simulink library "VMM_lib"  (Simulink 7.5)
settings: Solver=ode45  StartTime=0.0  StopTime=10.0  RelTol=1e-3
values from neighbouring files (symbols this model uses):
  pVMM_kmph_VehLgtSpdThd_C = Simulink.Parameter    [VMM_par.m]
  pVMM_s_EparkCheckTiOut_C = Simulink.Parameter    [VMM_par.m]
  pVMM_s_EparkShutdownTiOut_C = Simulink.Parameter    [VMM_par.m]
  pVMM_s_ShtdwnAckDly_C = Simulink.Parameter    [VMM_par.m]
  pVMM_s_ThermoShutdownTiOut_C = Simulink.Parameter    [VMM_par.m]
libraries: BaseOperationLib_Browser x15, PES_CZ_FAW x15, simulink x1
settings Model: Creator=wuaibin  LastModifiedBy=wuaibin

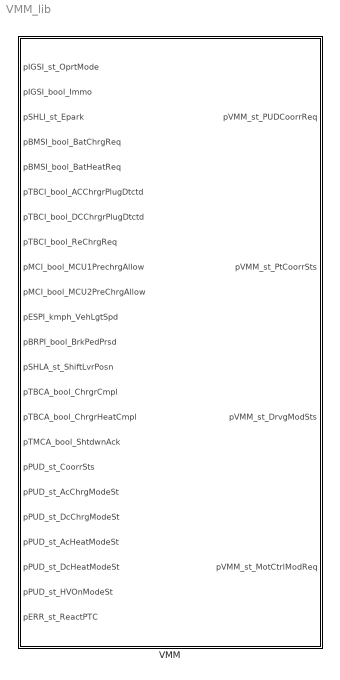
== system VMM_lib ==
  VMM : Subsystem  TreatAsAtomicUnit=on

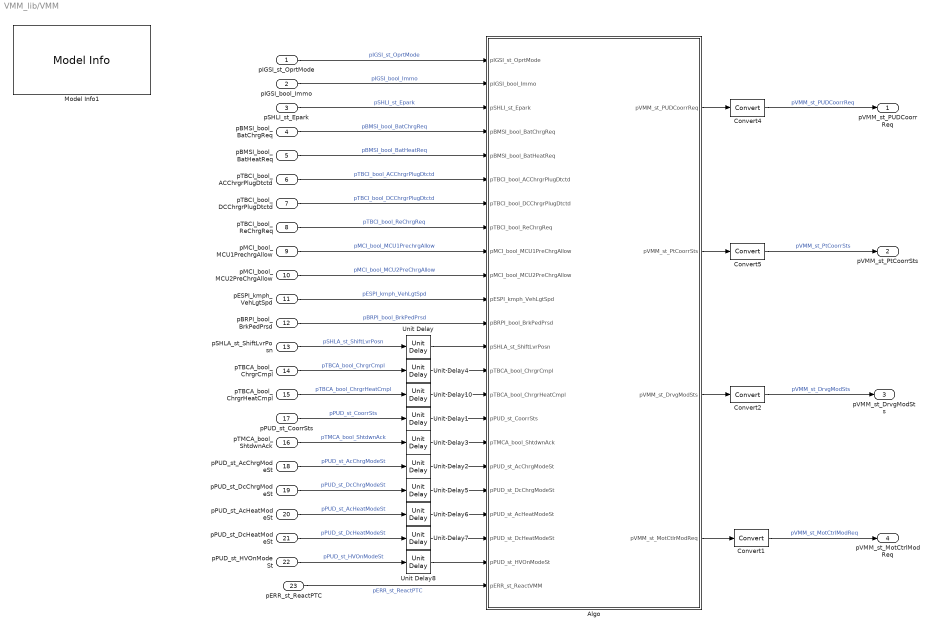
== system VMM_lib/VMM ==
  pIGSI_st_OprtMode : Inport
  pIGSI_bool_Immo : Inport  Port=2
  pSHLI_st_Epark : Inport  Port=3
  pBMSI_bool_BatChrgReq : Inport  Port=4
  pBMSI_bool_BatHeatReq : Inport  Port=5
  pTBCI_bool_ACChrgrPlugDtctd : Inport  Port=6
  pTBCI_bool_DCChrgrPlugDtctd : Inport  Port=7
  pTBCI_bool_ReChrgReq : Inport  Port=8
  pMCI_bool_MCU1PrechrgAllow : Inport  Port=9
  pMCI_bool_MCU2PreChrgAllow : Inport  Port=10
  pESPI_kmph_VehLgtSpd : Inport  Port=11
  pBRPI_bool_BrkPedPrsd : Inport  Port=12
  pSHLA_st_ShiftLvrPosn : Inport  Port=13
  pTBCA_bool_ChrgrCmpl : Inport  Port=14
  pTBCA_bool_ChrgrHeatCmpl : Inport  Port=15
  pTMCA_bool_ShtdwnAck : Inport  Port=16
  pPUD_st_CoorrSts : Inport  Port=17
  pPUD_st_AcChrgModeSt : Inport  Port=18
  pPUD_st_DcChrgModeSt : Inport  Port=19
  pPUD_st_AcHeatModeSt : Inport  Port=20
  pPUD_st_DcHeatModeSt : Inport  Port=21
  pPUD_st_HVOnModeSt : Inport  Port=22
  pERR_st_ReactPTC : Inport  Port=23
  Algo : Subsystem
  Convert{1..2,4..5} (4 alike) : DataTypeConversion  OutDataType=fixdt(1, 16)  OutScaling=2^0
  Model Info1 : simulink/Model-Wide Utilities/Model Info  SystemSampleTime=-1  InitialBlockCM=None  BlockCM=None  Frame=on  DisplayStringWithTags=Model Info\nCreated: %<Created>\nCreator: wuaibin  HorizontalTextAlignment=Center  LeftAlignmentValue=0.5  SourceBlockDiagram=untitled  TagMaxNumber=20
  Unit Delay{,1..8,10} (10 alike) : BaseOperationLib_Browser/Discrete Unchanged /Unit Delay  X0=0  SampleTime=-1
  pVMM_st_PUDCoorrReq : Outport
  pVMM_st_PtCoorrSts : Outport  Port=2
  pVMM_st_DrvgModSts : Outport  Port=3
  pVMM_st_MotCtrlModReq : Outport  Port=4
  wires:
  pTBCI_bool_ReChrgReq/1 -> Algo/8(pTBCI_bool_ReChrgReq)  "pTBCI_bool_ReChrgReq"
  Unit Delay10/1 -> Algo/15(pTBCA_bool_ChrgrHeatCmpl)
  pTBCA_bool_ChrgrHeatCmpl/1 -> Unit Delay10/1  "pTBCA_bool_ChrgrHeatCmpl"
  pMCI_bool_MCU2PreChrgAllow/1 -> Algo/10(pMCI_bool_MCU2PreChrgAllow)  "pMCI_bool_MCU2PreChrgAllow"
  Algo/4(pVMM_st_MotCtlrModReq) -> Convert1/1
  Convert1/1 -> pVMM_st_MotCtrlModReq/1  "pVMM_st_MotCtrlModReq"
  pMCI_bool_MCU1PrechrgAllow/1 -> Algo/9(pMCI_bool_MCU1PreChrgAllow)  "pMCI_bool_MCU1PrechrgAllow"
  Algo/1(pVMM_st_PUDCoorrReq) -> Convert4/1
  Algo/2(pVMM_st_PtCoorrSts) -> Convert5/1
  Algo/3(pVMM_st_DrvgModSts) -> Convert2/1
  pERR_st_ReactPTC/1 -> Algo/23(pERR_st_ReactVMM)  "pERR_st_ReactPTC"
  Unit Delay8/1 -> Algo/22(pPUD_st_HVOnModeSt)
  Unit Delay7/1 -> Algo/21(pPUD_st_DcHeatModeSt)
  Unit Delay6/1 -> Algo/20(pPUD_st_AcHeatModeSt)
  Unit Delay5/1 -> Algo/19(pPUD_st_DcChrgModeSt)
  Unit Delay2/1 -> Algo/18(pPUD_st_AcChrgModeSt)
  Unit Delay3/1 -> Algo/17(pTMCA_bool_ShtdwnAck)
  Unit Delay1/1 -> Algo/16(pPUD_st_CoorrSts)
  Unit Delay4/1 -> Algo/14(pTBCA_bool_ChrgrCmpl)
  Unit Delay/1 -> Algo/13(pSHLA_st_ShiftLvrPosn)
  pBRPI_bool_BrkPedPrsd/1 -> Algo/12(pBRPI_bool_BrkPedPrsd)  "pBRPI_bool_BrkPedPrsd"
  pESPI_kmph_VehLgtSpd/1 -> Algo/11(pESPI_kmph_VehLgtSpd)  "pESPI_kmph_VehLgtSpd"
  pTBCI_bool_DCChrgrPlugDtctd/1 -> Algo/7(pTBCI_bool_DCChrgrPlugDtctd)  "pTBCI_bool_DCChrgrPlugDtctd"
  pTBCI_bool_ACChrgrPlugDtctd/1 -> Algo/6(pTBCI_bool_ACChrgrPlugDtctd)  "pTBCI_bool_ACChrgrPlugDtctd"
  pBMSI_bool_BatHeatReq/1 -> Algo/5(pBMSI_bool_BatHeatReq)  "pBMSI_bool_BatHeatReq"
  pBMSI_bool_BatChrgReq/1 -> Algo/4(pBMSI_bool_BatChrgReq)  "pBMSI_bool_BatChrgReq"
  pSHLI_st_Epark/1 -> Algo/3(pSHLI_st_Epark)  "pSHLI_st_Epark"
  pIGSI_bool_Immo/1 -> Algo/2(pIGSI_bool_Immo)  "pIGSI_bool_Immo"
  pIGSI_st_OprtMode/1 -> Algo/1(pIGSI_st_OprtMode)  "pIGSI_st_OprtMode"
  Convert2/1 -> pVMM_st_DrvgModSts/1  "pVMM_st_DrvgModSts"
  pPUD_st_HVOnModeSt/1 -> Unit Delay8/1  "pPUD_st_HVOnModeSt"
  pPUD_st_DcHeatModeSt/1 -> Unit Delay7/1  "pPUD_st_DcHeatModeSt"
  pPUD_st_AcHeatModeSt/1 -> Unit Delay6/1  "pPUD_st_AcHeatModeSt"
  pPUD_st_DcChrgModeSt/1 -> Unit Delay5/1  "pPUD_st_DcChrgModeSt"
  pPUD_st_AcChrgModeSt/1 -> Unit Delay2/1  "pPUD_st_AcChrgModeSt"
  pTBCA_bool_ChrgrCmpl/1 -> Unit Delay4/1  "pTBCA_bool_ChrgrCmpl"
  pTMCA_bool_ShtdwnAck/1 -> Unit Delay3/1  "pTMCA_bool_ShtdwnAck"
  Convert5/1 -> pVMM_st_PtCoorrSts/1  "pVMM_st_PtCoorrSts"
  Convert4/1 -> pVMM_st_PUDCoorrReq/1  "pVMM_st_PUDCoorrReq"
  pPUD_st_CoorrSts/1 -> Unit Delay1/1  "pPUD_st_CoorrSts"
  pSHLA_st_ShiftLvrPosn/1 -> Unit Delay/1  "pSHLA_st_ShiftLvrPosn"

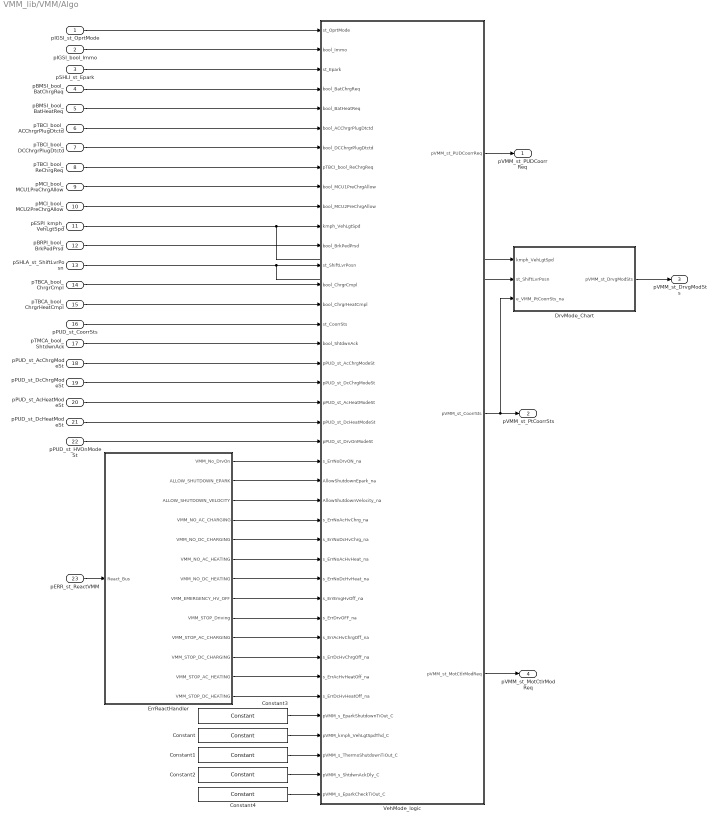
== system VMM_lib/VMM/Algo ==
  pIGSI_st_OprtMode : Inport
  pIGSI_bool_Immo : Inport  Port=2
  pSHLI_st_Epark : Inport  Port=3
  pBMSI_bool_BatChrgReq : Inport  Port=4
  pBMSI_bool_BatHeatReq : Inport  Port=5
  pTBCI_bool_ACChrgrPlugDtctd : Inport  Port=6
  pTBCI_bool_DCChrgrPlugDtctd : Inport  Port=7
  pTBCI_bool_ReChrgReq : Inport  Port=8
  pMCI_bool_MCU1PreChrgAllow : Inport  Port=9
  pMCI_bool_MCU2PreChrgAllow : Inport  Port=10
  pESPI_kmph_VehLgtSpd : Inport  Port=11
  pBRPI_bool_BrkPedPrsd : Inport  Port=12
  pSHLA_st_ShiftLvrPosn : Inport  Port=13
  pTBCA_bool_ChrgrCmpl : Inport  Port=14
  pTBCA_bool_ChrgrHeatCmpl : Inport  Port=15
  pPUD_st_CoorrSts : Inport  Port=16
  pTMCA_bool_ShtdwnAck : Inport  Port=17
  pPUD_st_AcChrgModeSt : Inport  Port=18
  pPUD_st_DcChrgModeSt : Inport  Port=19
  pPUD_st_AcHeatModeSt : Inport  Port=20
  pPUD_st_DcHeatModeSt : Inport  Port=21
  pPUD_st_HVOnModeSt : Inport  Port=22
  pERR_st_ReactVMM : Inport  Port=23
  Constant : BaseOperationLib_Browser/Sources&Sinks/Constant  Value=pVMM_kmph_VehLgtSpdThd_C  OutMin=[]  OutMax=[]  OutDataType=fixdt(1, 16)  ConRadixGroup=Use specified scaling  OutScaling=2^0  OutDataTypeStr=Inherit: Inherit from 'Constant value'
  Constant1 : BaseOperationLib_Browser/Sources&Sinks/Constant  Value=pVMM_s_ThermoShutdownTiOut_C  OutMin=[]  OutMax=[]  OutDataType=fixdt(1, 16)  ConRadixGroup=Use specified scaling  OutScaling=2^0  OutDataTypeStr=Inherit: Inherit from 'Constant value'
  Constant2 : BaseOperationLib_Browser/Sources&Sinks/Constant  Value=pVMM_s_ShtdwnAckDly_C  OutMin=[]  OutMax=[]  OutDataType=fixdt(1, 16)  ConRadixGroup=Use specified scaling  OutScaling=2^0  OutDataTypeStr=Inherit: Inherit from 'Constant value'
  Constant3 : BaseOperationLib_Browser/Sources&Sinks/Constant  Value=pVMM_s_EparkShutdownTiOut_C  OutMin=[]  OutMax=[]  OutDataType=fixdt(1, 16)  ConRadixGroup=Use specified scaling  OutScaling=2^0  OutDataTypeStr=Inherit: Inherit from 'Constant value'
  Constant4 : BaseOperationLib_Browser/Sources&Sinks/Constant  Value=pVMM_s_EparkCheckTiOut_C  OutMin=[]  OutMax=[]  OutDataType=fixdt(1, 16)  ConRadixGroup=Use specified scaling  OutScaling=2^0  OutDataTypeStr=Inherit: Inherit from 'Constant value'
  DrvMode_Chart : Stateflow chart  TreatAsAtomicUnit=on
  ErrReactHandler : Subsystem
  VehMode_logic : Stateflow chart  TreatAsAtomicUnit=on
  pVMM_st_PUDCoorrReq : Outport
  pVMM_st_PtCoorrSts : Outport  Port=2
  pVMM_st_DrvgModSts : Outport  Port=3
  pVMM_st_MotCtlrModReq : Outport  Port=4
  wires:
  Constant2/1 -> VehMode_logic/39(pVMM_s_ShtdwnAckDly_C)
  Constant1/1 -> VehMode_logic/38(pVMM_s_ThermoShutdownTiOut_C)
  Constant3/1 -> VehMode_logic/36(pVMM_s_EparkShutdownTiOut_C)
  Constant/1 -> VehMode_logic/37(pVMM_kmph_VehLgtSpdThd_C)
  pTBCI_bool_ReChrgReq/1 -> VehMode_logic/8(pTBCI_bool_ReChrgReq)
  pMCI_bool_MCU2PreChrgAllow/1 -> VehMode_logic/10(bool_MCU2PreChrgAllow)
  ErrReactHandler/13(VMM_STOP_DC_HEATING) -> VehMode_logic/35(s_ErrDcHvHeatOff_na)
  ErrReactHandler/12(VMM_STOP_AC_HEATING) -> VehMode_logic/34(s_ErrAcHvHeatOff_na)
  ErrReactHandler/11(VMM_STOP_DC_CHARGING) -> VehMode_logic/33(s_ErrDcHvChrgOff_na)
  ErrReactHandler/10(VMM_STOP_AC_CHARGING) -> VehMode_logic/32(s_ErrAcHvChrgOff_na)
  ErrReactHandler/9(VMM_STOP_Driving) -> VehMode_logic/31(s_ErrDrvOFF_na)
  VehMode_logic/2(pVMM_st_CoorrSts) -> DrvMode_Chart/3(e_VMM_PtCoorrSts_na), pVMM_st_PtCoorrSts/1
  pTBCA_bool_ChrgrHeatCmpl/1 -> VehMode_logic/15(bool_ChrgrHeatCmpl)
  pMCI_bool_MCU1PreChrgAllow/1 -> VehMode_logic/9(bool_MCU1PreChrgAllow)
  VehMode_logic/3(pVMM_st_MotCtlrModReq) -> pVMM_st_MotCtlrModReq/1
  pERR_st_ReactVMM/1 -> ErrReactHandler/1(React_Bus)
  ErrReactHandler/8(VMM_EMERGENCY_HV_OFF) -> VehMode_logic/30(s_ErrEmgHvOff_na)
  ErrReactHandler/7(VMM_NO_DC_HEATING) -> VehMode_logic/29(s_ErrNoDcHvHeat_na)
  ErrReactHandler/6(VMM_NO_AC_HEATING) -> VehMode_logic/28(s_ErrNoAcHvHeat_na)
  ErrReactHandler/5(VMM_NO_DC_CHARGING) -> VehMode_logic/27(s_ErrNoDcHvChrg_na)
  ErrReactHandler/4(VMM_NO_AC_CHARGING) -> VehMode_logic/26(s_ErrNoAcHvChrg_na)
  ErrReactHandler/3(ALLOW_SHUTDOWN_VELOCITY) -> VehMode_logic/25(AllowShutdownVelocity_na)
  ErrReactHandler/2(ALLOW_SHUTDOWN_EPARK) -> VehMode_logic/24(AllowShutdownEpark_na)
  ErrReactHandler/1(VMM_No_DrvOn) -> VehMode_logic/23(s_ErrNoDrvON_na)
  pPUD_st_HVOnModeSt/1 -> VehMode_logic/22(pPUD_st_DrvOnModeSt)
  pPUD_st_DcHeatModeSt/1 -> VehMode_logic/21(pPUD_st_DcHeatModeSt)
  pPUD_st_AcHeatModeSt/1 -> VehMode_logic/20(pPUD_st_AcHeatModeSt)
  pPUD_st_DcChrgModeSt/1 -> VehMode_logic/19(pPUD_st_DcChrgModeSt)
  pPUD_st_AcChrgModeSt/1 -> VehMode_logic/18(pPUD_st_AcChrgModeSt)
  pBMSI_bool_BatChrgReq/1 -> VehMode_logic/4(bool_BatChrgReq)
  VehMode_logic/1(pVMM_st_PUDCoorrReq) -> pVMM_st_PUDCoorrReq/1
  DrvMode_Chart/1(pVMM_st_DrvgModSts) -> pVMM_st_DrvgModSts/1
  pTMCA_bool_ShtdwnAck/1 -> VehMode_logic/17(bool_ShtdwnAck)
  pPUD_st_CoorrSts/1 -> VehMode_logic/16(st_CoorrSts)
  pTBCA_bool_ChrgrCmpl/1 -> VehMode_logic/14(bool_ChrgrCmpl)
  pSHLA_st_ShiftLvrPosn/1 -> VehMode_logic/13(st_ShiftLvrPosn), DrvMode_Chart/2(st_ShiftLvrPosn)
  pBRPI_bool_BrkPedPrsd/1 -> VehMode_logic/12(bool_BrkPedPrsd)
  pESPI_kmph_VehLgtSpd/1 -> VehMode_logic/11(kmph_VehLgtSpd), DrvMode_Chart/1(kmph_VehLgtSpd)
  pTBCI_bool_DCChrgrPlugDtctd/1 -> VehMode_logic/7(bool_DCChrgrPlugDtctd)
  pTBCI_bool_ACChrgrPlugDtctd/1 -> VehMode_logic/6(bool_ACChrgrPlugDtctd)
  pBMSI_bool_BatHeatReq/1 -> VehMode_logic/5(bool_BatHeatReq)
  pSHLI_st_Epark/1 -> VehMode_logic/3(st_Epark)
  pIGSI_bool_Immo/1 -> VehMode_logic/2(bool_Immo)
  pIGSI_st_OprtMode/1 -> VehMode_logic/1(st_OprtMode)
  Constant4/1 -> VehMode_logic/40(pVMM_s_EparkCheckTiOut_C)

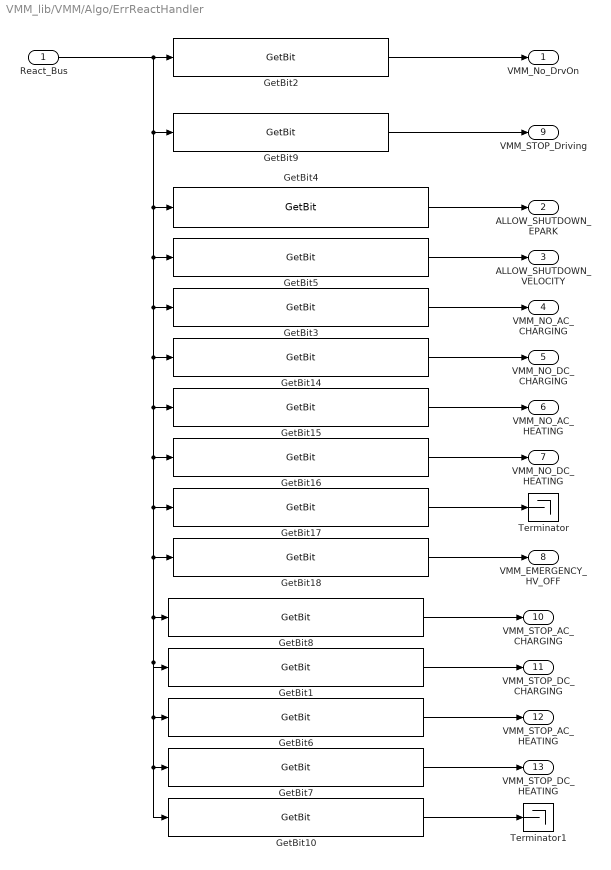
== system VMM_lib/VMM/Algo/ErrReactHandler ==
  React_Bus : Inport
  GetBit1 : PES_CZ_FAW/Discontinuities/GetBit  SystemSampleTime=-1  maska=FtlReactVMMTyp.VMM_STOP_DC_CHARGING
  GetBit10 : PES_CZ_FAW/Discontinuities/GetBit  SystemSampleTime=-1  maska=FtlReactVMMTyp.VMM_STOP_Rem_AC
  GetBit14 : PES_CZ_FAW/Discontinuities/GetBit  SystemSampleTime=-1  maska=FtlReactVMMTyp.VMM_NO_DC_CHARGING
  GetBit15 : PES_CZ_FAW/Discontinuities/GetBit  SystemSampleTime=-1  maska=FtlReactVMMTyp.VMM_NO_AC_HEATING
  GetBit16 : PES_CZ_FAW/Discontinuities/GetBit  SystemSampleTime=-1  maska=FtlReactVMMTyp.VMM_NO_DC_HEATING
  GetBit17 : PES_CZ_FAW/Discontinuities/GetBit  SystemSampleTime=-1  maska=FtlReactVMMTyp.VMM_NO_Rem_AC
  GetBit18 : PES_CZ_FAW/Discontinuities/GetBit  SystemSampleTime=-1  maska=FtlReactVMMTyp.VMM_EMERGENCY_HV_OFF
  GetBit2 : PES_CZ_FAW/Discontinuities/GetBit  SystemSampleTime=-1  maska=FtlReactVMMTyp.BLOCK_DRIVING_TRANS
  GetBit3 : PES_CZ_FAW/Discontinuities/GetBit  SystemSampleTime=-1  maska=FtlReactVMMTyp.VMM_NO_AC_CHARGING
  GetBit4 : PES_CZ_FAW/Discontinuities/GetBit  SystemSampleTime=-1  maska=FtlReactVMMTyp.ALLOW_SHUTDOWN_EPARK
  GetBit5 : PES_CZ_FAW/Discontinuities/GetBit  SystemSampleTime=-1  maska=FtlReactVMMTyp.ALLOW_SHUTDOWN_VELOCITY
  GetBit6 : PES_CZ_FAW/Discontinuities/GetBit  SystemSampleTime=-1  maska=FtlReactVMMTyp.VMM_STOP_AC_HEATING
  GetBit7 : PES_CZ_FAW/Discontinuities/GetBit  SystemSampleTime=-1  maska=FtlReactVMMTyp.VMM_STOP_DC_HEATING
  GetBit8 : PES_CZ_FAW/Discontinuities/GetBit  SystemSampleTime=-1  maska=FtlReactVMMTyp.VMM_STOP_AC_CHARGING
  GetBit9 : PES_CZ_FAW/Discontinuities/GetBit  SystemSampleTime=-1  maska=FtlReactVMMTyp.VMM_STOP_DRIVING
  Terminator : Terminator
  Terminator1 : Terminator
  VMM_No_DrvOn : Outport
  ALLOW_SHUTDOWN_EPARK : Outport  Port=2
  ALLOW_SHUTDOWN_VELOCITY : Outport  Port=3
  VMM_NO_AC_CHARGING : Outport  Port=4
  VMM_NO_DC_CHARGING : Outport  Port=5
  VMM_NO_AC_HEATING : Outport  Port=6
  VMM_NO_DC_HEATING : Outport  Port=7
  VMM_EMERGENCY_HV_OFF : Outport  Port=8
  VMM_STOP_Driving : Outport  Port=9
  VMM_STOP_AC_CHARGING : Outport  Port=10
  VMM_STOP_DC_CHARGING : Outport  Port=11
  VMM_STOP_AC_HEATING : Outport  Port=12
  VMM_STOP_DC_HEATING : Outport  Port=13
  wires:
  GetBit10/1 -> Terminator1/1
  GetBit9/1 -> VMM_STOP_Driving/1
  GetBit7/1 -> VMM_STOP_DC_HEATING/1
  GetBit6/1 -> VMM_STOP_AC_HEATING/1
  GetBit1/1 -> VMM_STOP_DC_CHARGING/1
  GetBit8/1 -> VMM_STOP_AC_CHARGING/1
  GetBit18/1 -> VMM_EMERGENCY_HV_OFF/1
  GetBit17/1 -> Terminator/1
  GetBit16/1 -> VMM_NO_DC_HEATING/1
  GetBit15/1 -> VMM_NO_AC_HEATING/1
  GetBit14/1 -> VMM_NO_DC_CHARGING/1
  GetBit3/1 -> VMM_NO_AC_CHARGING/1
  GetBit5/1 -> ALLOW_SHUTDOWN_VELOCITY/1
  GetBit4/1 -> ALLOW_SHUTDOWN_EPARK/1
  GetBit2/1 -> VMM_No_DrvOn/1
  React_Bus/1 -> GetBit9/1, GetBit10/1, GetBit7/1, GetBit6/1, GetBit1/1, GetBit8/1, GetBit18/1, GetBit17/1, GetBit16/1, GetBit15/1, GetBit14/1, GetBit3/1, GetBit5/1, GetBit4/1, GetBit2/1

== stateflow chart VMM/Algo/DrvMode_Chart ==
  state Drv
    state Driving
      en:
      pVMM_st_DrvgModSts = DrvgModStsTyp.DRV;
    state Creeping
      en:
      pVMM_st_DrvgModSts = DrvgModStsTyp.CREEP;
    (default) -> Creeping
    Creeping -> Driving : [((st_ShiftLvrPosn == ShiftLvrPosnTyp.SHL_D || ...
        | st_ShiftLvrPosn == ShiftLvrPosnTyp.SHL_R) && ...
        | kmph_VehLgtSpd >=p_PTC_VehSpdCreepThd_kmph)]
    Driving -> Creeping : [((st_ShiftLvrPosn == ShiftLvrPosnTyp.SHL_D || ...
        | st_ShiftLvrPosn == ShiftLvrPosnTyp.SHL_R) && ...
        | kmph_VehLgtSpd < p_PTC_VehSpdCreepThd_kmph)]
  state StandStill
    state Neutral
      en:
      pVMM_st_DrvgModSts = DrvgModStsTyp.NEUT;
    state Parking
      en:
      pVMM_st_DrvgModSts = DrvgModStsTyp.PRK;
    Neutral -> Parking : [st_ShiftLvrPosn == ShiftLvrPosnTyp.SHL_P]
    (default) -> Parking
    Parking -> Neutral : [st_ShiftLvrPosn == ShiftLvrPosnTyp.SHL_N]
  Drv -> Neutral [order 1] : [st_ShiftLvrPosn == ShiftLvrPosnTyp.SHL_N || ...
      | e_VMM_PtCoorrSts_na !=VMMCoorrStsTyp.VMM_Drv]
  Drv -> Parking [order 2] : [st_ShiftLvrPosn == SHL_P]
  (default) -> StandStill
  StandStill -> Drv : [(st_ShiftLvrPosn == ShiftLvrPosnTyp.SHL_D || ...
      | st_ShiftLvrPosn == ShiftLvrPosnTyp.SHL_R) && ...
      | e_VMM_PtCoorrSts_na ==VMMCoorrStsTyp.VMM_Drv]
  data: kmph_VehLgtSpd input double; pVMM_st_DrvgModSts output uint8; st_ShiftLvrPosn input double; e_VMM_PtCoorrSts_na input double; p_PTC_VehSpdCreepThd_kmph parameter double

== stateflow chart VMM/Algo/VehMode_logic ==
  state bool_DrvOffErrFlag = DrvErrOffFlag [function]
    (junction 138) -> (junction 140) : {
        | bool_DrvOffErrFlag = true;
        | }
    (junction 129) -> (junction 130) [order 1] : [s_ErrDrvOFF_na]
    (junction 131) -> (junction 133)
    (junction 132) -> (junction 131)
    (junction 129) -> (junction 131) [order 2] : {
        | bool_DrvOffErrFlag = false;
        | }
    (junction 130) -> (junction 132) : {
        | bool_DrvOffErrFlag = true;
        | }
    (junction 143) -> (junction 129) [order 2]
    (junction 143) -> (junction 138) [order 1] : [pVMM_st_CoorrSts != VMMCoorrStsTyp.VMM_Drv && ...
        | st_Epark == EparkModTyp.Epk_Failed]
    (junction 140) -> (junction 132)
    (default) -> (junction 143)
  state bool_DCHeatErrFlag = DCHeatErrFlag [function]
    (junction 103) -> (junction 186)
    (junction 184) -> (junction 182) [order 2] : {
        | bool_DCHeatErrFlag = false;
        | }
    (default) -> (junction 187)
    (junction 93) -> (junction 103) : {
        | bool_DCHeatErrFlag = true;
        | }
    (junction 187) -> (junction 93) [order 1] : [pPUD_st_DcHeatModeSt == DCHeatModeTyp.PUD_DCHeat_Err]
    (junction 185) -> (junction 186) : {
        | bool_DCHeatErrFlag = true;
        | }
    (junction 182) -> (junction 183)
    (junction 187) -> (junction 184) [order 2]
    (junction 186) -> (junction 182)
    (junction 184) -> (junction 185) [order 1] : [s_ErrDcHvHeatOff_na]
  state bool_ACChrgFlag = ACChrgFlag [function]
    (default) -> (junction 100)
    (junction 100) -> (junction 102) [order 1] : [bool_ACChrgrPlugDtctd && ...
        | bool_BatChrgReq == true && ...
        | st_ShiftLvrPosn == ShiftLvrPosnTyp.SHL_P && ...
        | bool_MCU1PreChrgAllow == true && ...
        | bool_MCU2PreChrgAllow == true && ...
        | !s_ErrNoAcHvChrg_na]
    (junction 105) -> (junction 120)
    (junction 102) -> (junction 105) : {
        | bool_ACChrgFlag = true;
        | }
    (junction 120) -> (junction 119)
    (junction 100) -> (junction 120) [order 2] : {
        | bool_ACChrgFlag = false;
        | }
  state Norm
    state DCHeat
      state DCHeating
        entry:
        pVMM_st_CoorrSts =VMMCoorrStsTyp.VMM_DCHeating;
      state DCHeat
        entry:
        pVMM_st_MotCtlrModReq = MotCtrlModTyp.MTC_INIT;
        pVMM_st_PUDCoorrReq= PUDCoorrStsTyp.PUD_DCHeatOn;
        pVMM_st_CoorrSts =VMMCoorrStsTyp.VMM_DCHeatOn;
      Norm.DCHeat.DCHeat -> DCHeating : [pPUD_st_DcHeatModeSt == DCHeatModeTyp.PUD_DCHeat_On]
      (default) -> Norm.DCHeat.DCHeat
    state KeyOn
      entry:
      pVMM_st_CoorrSts =VMMCoorrStsTyp.VMM_KeyOn;
      pVMM_st_MotCtlrModReq = MotCtrlModTyp.MTC_INIT;
    state Drv
      state DrvOn_Ok
        en:
        pVMM_st_CoorrSts = VMMCoorrStsTyp.VMM_DrvOnOk;
        pVMM_st_MotCtlrModReq = MotCtrlModTyp.MTC_STANDBY;
      state Drv_Err
        en:
        pVMM_st_CoorrSts = VMMCoorrStsTyp.VMM_DrvErr;
        pVMM_st_PUDCoorrReq = PUDCoorrStsTyp.PUD_DrvErr;
        pVMM_st_MotCtlrModReq = MotCtrlModTyp.MTC_STOP;
        exit:
        bool_restart = false;
        Drv_Err -> Drv_Err [order 1] : [st_OprtMode <= OperModTyp.CL15]
            | {bool_restart = true;}
      state Drv
        en:
        pVMM_st_CoorrSts = VMMCoorrStsTyp.VMM_Drv;
        pVMM_st_MotCtlrModReq = MotCtrlModTyp.MTC_TQ_IDLE;
      state DrvOn_Init
        en:
        pVMM_st_CoorrSts = VMMCoorrStsTyp.VMM_DrvOn;
        pVMM_st_PUDCoorrReq = PUDCoorrStsTyp.PUD_DrvOn;
        pVMM_st_MotCtlrModReq = MotCtrlModTyp.MTC_INIT;
      Drv_Err -> DrvOn_Init [order 1] : [st_OprtMode == OperModTyp.CL50 && ...
          | DrvFlag() && ...
          | bool_restart == true]
      (default) -> DrvOn_Init
      DrvOn_Init -> DrvOn_Ok [order 1] : [pPUD_st_DrvOnModeSt == PUDCoorrStsTyp.PUD_DrvOn]
      DrvOn_Ok -> Drv_Err [order 2] : [after(pVMM_s_EparkCheckTiOut_C,sec)]
      DrvOn_Ok -> Norm.Drv.Drv [order 1] : [st_Epark == EparkModTyp.Epk_Success]
      DrvOn_Init -> Drv_Err [order 2] : [pPUD_st_DrvOnModeSt == DrvOnModeTyp.PUD_DrvOn_Err || ...
          | s_ErrNoDrvON_na ]
    state ACChrg
      state Chrg
        entry:
        pVMM_st_MotCtlrModReq = MotCtrlModTyp.MTC_INIT;
        pVMM_st_PUDCoorrReq= PUDCoorrStsTyp.PUD_ACChrgOn;
        pVMM_st_CoorrSts =VMMCoorrStsTyp.VMM_ACChrgOn;
      state ACCharging
        entry:
        pVMM_st_CoorrSts =VMMCoorrStsTyp.VMM_ACCharging;
      Chrg -> ACCharging : [pPUD_st_AcChrgModeSt == ACChrgModeTyp.PUD_ACChrg_On]
      (default) -> Chrg
    state Init
      en:
      pVMM_st_CoorrSts =VMMCoorrStsTyp.VMM_Init;
      pVMM_st_MotCtlrModReq = MotCtrlModTyp.MTC_INIT;
    state Shtdwn
      en:
      pVMM_st_CoorrSts =VMMCoorrStsTyp.VMM_ShtDwn;
      state Check_P
      state Shutdown_ack
        en:
        pVMM_st_CoorrSts =VMMCoorrStsTyp.VMM_LvPwrOff;
      state Thermo_shutdown
      state PUD_Off
        en:
        pVMM_st_PUDCoorrReq = PUDCoorrStsTyp.PUD_HVOFF;
        pVMM_st_MotCtlrModReq = MotCtrlModTyp.MTC_SHUTDOWN;
      Norm.Shtdwn.Check_P -> Norm.Shtdwn.Shutdown_ack [order 1] : [st_ShiftLvrPosn == ShiftLvrPosnTyp.SHL_P || ...
          | AllowShutdownEpark_na == true]
      (default) -> PUD_Off
      Norm.Shtdwn.Check_P -> Norm.Shtdwn.Shutdown_ack [order 2] : after(pVMM_s_EparkShutdownTiOut_C, sec)
      PUD_Off -> Norm.Shtdwn.Thermo_shutdown : [st_CoorrSts == PUDCoorrStsTyp.PUD_HVOFF_OK]
      Norm.Shtdwn.Thermo_shutdown -> Norm.Shtdwn.Check_P [order 1] : [bool_ShtdwnAck == true]
      Norm.Shtdwn.Thermo_shutdown -> Norm.Shtdwn.Check_P [order 2] : after(pVMM_s_ThermoShutdownTiOut_C, sec)
    state ACHeat
      state ACHeat
        entry:
        pVMM_st_PUDCoorrReq= PUDCoorrStsTyp.PUD_ACHeatOn;
        pVMM_st_MotCtlrModReq = MotCtrlModTyp.MTC_INIT;
        pVMM_st_CoorrSts =VMMCoorrStsTyp.VMM_ACHeatOn;
      state ACHeating
        entry:
        pVMM_st_CoorrSts =VMMCoorrStsTyp.VMM_ACHeating;
      Norm.ACHeat.ACHeat -> ACHeating : [pPUD_st_AcHeatModeSt == ACHeatModeTyp.PUD_ACHeat_On]
      (default) -> Norm.ACHeat.ACHeat
    state DCChrg
      state DCChrgOn
        entry:
        pVMM_st_MotCtlrModReq = MotCtrlModTyp.MTC_INIT;
        pVMM_st_PUDCoorrReq= PUDCoorrStsTyp.PUD_DCChrgOn;
        pVMM_st_CoorrSts =VMMCoorrStsTyp.VMM_DCChrgOn;
      state DCCharging
        entry:
        pVMM_st_CoorrSts =VMMCoorrStsTyp.VMM_DCCharging;
      DCChrgOn -> DCCharging : [pPUD_st_DcChrgModeSt == DCChrgModeTyp.PUD_DCChrg_On]
      (default) -> DCChrgOn
    Norm.Drv -> Shtdwn : [st_OprtMode < OperModTyp.CL15 || ...
        | DrvShtDwnFlag() || ...
        | DrvErrOffFlag()]
    Shtdwn -> ACChrg [order 2] : [st_OprtMode < OperModTyp.CL15 && ...
        | ACChrgFlag() && ...
        | !ACChrgErrFlag()]
    ACChrg -> Shtdwn : [ACChrgShtDwnFlag() || ...
        | ACChrgErrFlag()]
    Shtdwn -> DCChrg [order 3] : [st_OprtMode < OperModTyp.CL15 && ...
        | DCChrgFlag() && ...
        | !DCChrgErrFlag()]
    KeyOn -> Norm.Drv [order 2] : [st_OprtMode == OperModTyp.CL50 && ...
        | DrvFlag()]
    Shtdwn -> KeyOn [order 1] : [st_OprtMode >= OperModTyp.CL15 && ...
        | !DrvShtDwnFlag() && ...
        | !DrvErrOffFlag()]
    KeyOn -> Shtdwn [order 1] : [st_OprtMode < OperModTyp.CL15]
    Init -> KeyOn [order 1] : [st_OprtMode >= OperModTyp.CL15]
    Init -> ACChrg [order 2] : [st_OprtMode < OperModTyp.CL15 && ...
        | ACChrgFlag()]
    Init -> Shtdwn [order 4] : [after(pVMM_s_ShtdwnAckDly_C,sec)]
    (default) -> Init
    Norm.DCHeat -> Shtdwn : [DCHeatShtDwnFlag() || ...
        | DCHeatErrFlag()]
    DCChrg -> Shtdwn : [DCChrgShtDwnFlag() || ...
        | DCChrgErrFlag()]
    Init -> DCChrg [order 3] : [st_OprtMode < OperModTyp.CL15 && ...
        | DCChrgFlag() ]
    Shtdwn -> Norm.ACHeat [order 5] : [st_OprtMode < OperModTyp.CL15 && ...
        | ACHeatFlag() && ...
        | !ACHeatErrFlag()]
    Norm.ACHeat -> Shtdwn : [ACHeatShtDwnFlag() || ...
        | ACHeatErrFlag()]
    Init -> Norm.ACHeat [order 6] : [st_OprtMode < OperModTyp.CL15 && ...
        | ACHeatFlag()]
    Shtdwn -> Norm.DCHeat [order 4] : [st_OprtMode < OperModTyp.CL15 && ...
        | DCHeatFlag() && ...
        | !DCHeatErrFlag()]
    Init -> Norm.DCHeat [order 5] : [st_OprtMode < OperModTyp.CL15 && ...
        | DCHeatFlag() ]
  state SafeMode
    en:
    pVMM_st_CoorrSts =VMMCoorrStsTyp.VMM_SafeMode;
    state Shutdown_ack
      en:
      pVMM_st_CoorrSts =VMMCoorrStsTyp.VMM_LvPwrOff;
    state Egc_Off
      en:
      pVMM_st_PUDCoorrReq = PUDCoorrStsTyp.PUD_EmgHVOFF;
      pVMM_st_MotCtlrModReq = MotCtrlModTyp.MTC_SHUTDOWN;
    state Check_KeyOFF
    state Thermo_shutdown
    state Check_P
    (default) -> Egc_Off
    Egc_Off -> Check_KeyOFF : [st_CoorrSts == PUDCoorrStsTyp.PUD_EmgHVOFF_OK]
    Check_KeyOFF -> SafeMode.Thermo_shutdown : [st_OprtMode < OperModTyp.CL15]
    SafeMode.Thermo_shutdown -> SafeMode.Check_P [order 1] : [bool_ShtdwnAck == true]
    SafeMode.Thermo_shutdown -> SafeMode.Check_P [order 2] : after(pVMM_s_ThermoShutdownTiOut_C, sec)
    SafeMode.Check_P -> SafeMode.Shutdown_ack [order 1] : [st_ShiftLvrPosn == ShiftLvrPosnTyp.SHL_P || ...
        | AllowShutdownEpark_na == true]
    SafeMode.Check_P -> SafeMode.Shutdown_ack [order 2] : after(pVMM_s_EparkShutdownTiOut_C, sec)
  state bool_DrvFlag = DrvFlag [function]
    (junction 98) -> (junction 101)
    (default) -> (junction 96)
    (junction 99) -> (junction 98)
    (junction 96) -> (junction 98) [order 2] : {
        | bool_DrvFlag = false;
        | }
    (junction 97) -> (junction 99) : {
        | bool_DrvFlag = true;
        | }
    (junction 96) -> (junction 97) [order 1] : [!bool_ACChrgrPlugDtctd && ...
        | !bool_DCChrgrPlugDtctd && ...
        | (st_ShiftLvrPosn == ShiftLvrPosnTyp.SHL_P || ...
        | st_ShiftLvrPosn == ShiftLvrPosnTyp.SHL_N) && ...
        | bool_BrkPedPrsd && ...
        | bool_MCU1PreChrgAllow == true && ...
        | bool_MCU2PreChrgAllow == true && ...
        | bool_Immo == ImmoModTyp.Immo_Success && ...
        | st_Epark != EparkModTyp.Epk_Failed && ...
        | !s_ErrNoDrvON_na]
  state bool_DrvShtDwnFlag = DrvShtDwnFlag [function]
    (default) -> (junction 76)
    (junction 76) -> (junction 82) [order 2] : {
        | bool_DrvShtDwnFlag = false;
        | }
    (junction 76) -> (junction 78) [order 1] : [(bool_ACChrgrPlugDtctd == true || bool_DCChrgrPlugDtctd == true ) && ...
        | (kmph_VehLgtSpd < pVMM_kmph_VehLgtSpdThd_C || AllowShutdownVelocity_na)]
    (junction 78) -> (junction 84) : {
        | bool_DrvShtDwnFlag = true;
        | }
    (junction 82) -> (junction 85)
    (junction 84) -> (junction 82)
  state bool_ACChrgErrFlag = ACChrgErrFlag [function]
    (default) -> (junction 77)
    (junction 107) -> (junction 104)
    (junction 106) -> (junction 107)
    (junction 110) -> (junction 106)
    (junction 116) -> (junction 106) : {
        | bool_ACChrgErrFlag = true;
        | }
    (junction 117) -> (junction 107) [order 2] : {
        | bool_ACChrgErrFlag = false;
        | }
    (junction 117) -> (junction 116) [order 1] : [s_ErrAcHvChrgOff_na]
    (junction 118) -> (junction 110) : {
        | bool_ACChrgErrFlag = true;
        | }
    (junction 77) -> (junction 117) [order 2]
    (junction 77) -> (junction 118) [order 1] : [pPUD_st_AcChrgModeSt == ACChrgModeTyp.PUD_ACChrg_Err  && ...
        | pTBCI_bool_ReChrgReq == false]
  state bool_ACChrgShtDwnFlag = ACChrgShtDwnFlag [function]
    (junction 73) -> (junction 87) : {
        | bool_ACChrgShtDwnFlag = true;
        | }
    (junction 86) -> (junction 94) [order 2]
    (junction 86) -> (junction 73) [order 1] : [!bool_ACChrgrPlugDtctd]
    (junction 127) -> (junction 145) [order 2] : {
        | bool_ACChrgShtDwnFlag = false;
        | }
    (junction 94) -> (junction 127) [order 2]
    (junction 92) -> (junction 122) : {
        | bool_ACChrgShtDwnFlag = true;
        | }
    (junction 94) -> (junction 92) [order 1] : [bool_BatChrgReq == false]
    (junction 87) -> (junction 122)
    (default) -> (junction 86)
    (junction 145) -> (junction 144)
    (junction 122) -> (junction 147)
    (junction 127) -> (junction 146) [order 1] : [bool_ChrgrCmpl]
    (junction 146) -> (junction 147) : {
        | bool_ACChrgShtDwnFlag = true;
        | }
    (junction 147) -> (junction 145)
  state bool_DCChrgShtDwnFlag = DCChrgShtDwnFlag [function]
    (junction 154) -> (junction 142) [order 2] : {
        | bool_DCChrgShtDwnFlag = false;
        | }
    (junction 154) -> (junction 155) [order 1] : [bool_ChrgrCmpl]
    (junction 142) -> (junction 134)
    (junction 135) -> (junction 136)
    (junction 136) -> (junction 137)
    (junction 137) -> (junction 142)
    (junction 155) -> (junction 137) : {
        | bool_DCChrgShtDwnFlag = true;
        | }
    (default) -> (junction 150)
    (junction 150) -> (junction 151) [order 1] : [!bool_DCChrgrPlugDtctd]
    (junction 150) -> (junction 152) [order 2]
    (junction 151) -> (junction 135) : {
        | bool_DCChrgShtDwnFlag = true;
        | }
    (junction 152) -> (junction 153) [order 1] : [bool_BatChrgReq == false]
    (junction 153) -> (junction 136) : {
        | bool_DCChrgShtDwnFlag = true;
        | }
    (junction 152) -> (junction 154) [order 2]
  state bool_DCChrgFlag = DCChrgFlag [function]
    (junction 72) -> (junction 74) [order 2] : {
        | bool_DCChrgFlag = false;
        | }
    (junction 74) -> (junction 141)
    (default) -> (junction 72)
    (junction 123) -> (junction 81) : {
        | bool_DCChrgFlag = true;
        | }
    (junction 81) -> (junction 74)
    (junction 72) -> (junction 123) [order 1] : [bool_DCChrgrPlugDtctd && ...
        | bool_BatChrgReq == true && ...
        | st_ShiftLvrPosn == ShiftLvrPosnTyp.SHL_P && ...
        | bool_MCU1PreChrgAllow == true && ...
        | bool_MCU2PreChrgAllow == true && ...
        | !s_ErrNoDcHvChrg_na]
  state bool_DCChrgErrFlag = DCChrgErrFlag [function]
    (junction 91) -> (junction 80)
    (junction 89) -> (junction 91)
    (junction 124) -> (junction 89)
    (junction 125) -> (junction 89) : {
        | bool_DCChrgErrFlag = true;
        | }
    (junction 126) -> (junction 91) [order 2] : {
        | bool_DCChrgErrFlag = false;
        | }
    (junction 126) -> (junction 125) [order 1] : [s_ErrDcHvChrgOff_na]
    (junction 139) -> (junction 124) : {
        | bool_DCChrgErrFlag = true;
        | }
    (junction 75) -> (junction 126) [order 2]
    (junction 75) -> (junction 139) [order 1] : [pPUD_st_DcChrgModeSt == DCChrgModeTyp.PUD_DCChrg_Err]
    (default) -> (junction 75)
  state bool_ACHeatFlag = ACHeatFlag [function]
    (junction 83) -> (junction 88)
    (junction 88) -> (junction 108)
    (junction 90) -> (junction 83) : {
        | bool_ACHeatFlag = true;
        | }
    (junction 128) -> (junction 88) [order 2] : {
        | bool_ACHeatFlag = false;
        | }
    (junction 128) -> (junction 90) [order 1] : [bool_ACChrgrPlugDtctd && ...
        | bool_BatHeatReq == true && ...
        | st_ShiftLvrPosn == ShiftLvrPosnTyp.SHL_P && ...
        | bool_MCU1PreChrgAllow == true && ...
        | bool_MCU2PreChrgAllow == true && ...
        | !s_ErrNoAcHvHeat_na]
    (default) -> (junction 128)
  state bool_DCHeatFlag = DCHeatFlag [function]
    (default) -> (junction 112)
    (junction 114) -> (junction 111) : {
        | bool_DCHeatFlag = true;
        | }
    (junction 112) -> (junction 109) [order 2] : {
        | bool_DCHeatFlag = false;
        | }
    (junction 111) -> (junction 109)
    (junction 112) -> (junction 114) [order 1] : [bool_DCChrgrPlugDtctd && ...
        | bool_BatHeatReq == true && ...
        | st_ShiftLvrPosn == ShiftLvrPosnTyp.SHL_P && ...
        | bool_MCU1PreChrgAllow == true && ...
        | bool_MCU2PreChrgAllow == true && ...
        | !s_ErrNoDcHvHeat_na]
    (junction 109) -> (junction 113)
  state bool_ACHeatErrFlag = ACHeatErrFlag [function]
    (junction 95) -> (junction 79) [order 1] : [pPUD_st_AcHeatModeSt == ACHeatModeTyp.PUD_ACHeat_Err  && ...
        | pTBCI_bool_ReChrgReq == false]
    (default) -> (junction 95)
    (junction 159) -> (junction 160)
    (junction 161) -> (junction 159)
    (junction 163) -> (junction 159) : {
        | bool_ACHeatErrFlag = true;
        | }
    (junction 173) -> (junction 160) [order 2] : {
        | bool_ACHeatErrFlag = false;
        | }
    (junction 173) -> (junction 163) [order 1] : [s_ErrAcHvHeatOff_na]
    (junction 160) -> (junction 158)
    (junction 79) -> (junction 161) : {
        | bool_ACHeatErrFlag = true;
        | }
    (junction 95) -> (junction 173) [order 2]
  state bool_ACHeatShtDwnFlag = ACHeatShtDwnFlag [function]
    (junction 148) -> (junction 115)
    (junction 157) -> (junction 162)
    (junction 167) -> (junction 162) : {
        | bool_ACHeatShtDwnFlag = true;
        | }
    (junction 149) -> (junction 148) [order 2] : {
        | bool_ACHeatShtDwnFlag = false;
        | }
    (junction 166) -> (junction 149) [order 2]
    (junction 166) -> (junction 167) [order 1] : [bool_BatHeatReq == false]
    (junction 156) -> (junction 121) : {
        | bool_ACHeatShtDwnFlag = true;
        | }
    (junction 149) -> (junction 156) [order 1] : [ bool_ChrgrHeatCmpl]
    (junction 162) -> (junction 121)
    (junction 121) -> (junction 148)
    (default) -> (junction 164)
    (junction 164) -> (junction 165) [order 1] : [!bool_ACChrgrPlugDtctd]
    (junction 164) -> (junction 166) [order 2]
    (junction 165) -> (junction 157) : {
        | bool_ACHeatShtDwnFlag = true;
        | }
  state bool_DCHeatShtDwnFlag = DCHeatShtDwnFlag [function]
    (default) -> (junction 168)
    (junction 168) -> (junction 169) [order 1] : [!bool_DCChrgrPlugDtctd]
    (junction 168) -> (junction 170) [order 2]
    (junction 169) -> (junction 180) : {
        | bool_DCHeatShtDwnFlag = true;
        | }
    (junction 170) -> (junction 171) [order 1] : [bool_BatHeatReq == false]
    (junction 171) -> (junction 179) : {
        | bool_DCHeatShtDwnFlag = true;
        | }
    (junction 170) -> (junction 172) [order 2]
    (junction 172) -> (junction 174) [order 2]
    (junction 172) -> (junction 175) [order 1] : [bool_ChrgrHeatCmpl]
    (junction 175) -> (junction 178) : {
        | bool_DCHeatShtDwnFlag = true;
        | }
    (junction 174) -> (junction 176) : {
        | bool_DCHeatShtDwnFlag = false;
        | }
    (junction 177) -> (junction 176)
    (junction 178) -> (junction 177)
    (junction 179) -> (junction 178)
    (junction 180) -> (junction 179)
    (junction 176) -> (junction 181)
  (default) -> Norm
  Norm -> SafeMode : [s_ErrEmgHvOff_na]
  data: bool_DrvOffErrFlag function_output double; bool_DCHeatErrFlag function_output double; bool_ACChrgFlag function_output double; bool_DrvFlag function_output double; bool_DrvShtDwnFlag function_output double; bool_ACChrgErrFlag function_output double; bool_ACChrgShtDwnFlag function_output double; bool_DCChrgShtDwnFlag function_output double; bool_DCChrgFlag function_output double; bool_DCChrgErrFlag function_output double; bool_ACHeatFlag function_output double; bool_DCHeatFlag function_output double; bool_ACHeatErrFlag function_output double; bool_ACHeatShtDwnFlag function_output double; bool_DCHeatShtDwnFlag function_output double; st_OprtMode input uint8; bool_Immo input double; st_Epark input double; bool_BatChrgReq input double; bool_BatHeatReq input double; bool_ACChrgrPlugDtctd input double; bool_DCChrgrPlugDtctd input double; pTBCI_bool_ReChrgReq input double; bool_MCU1PreChrgAllow input double; bool_MCU2PreChrgAllow input double; kmph_VehLgtSpd input double; bool_BrkPedPrsd input double; st_ShiftLvrPosn input double; bool_ChrgrCmpl input boolean; bool_ChrgrHeatCmpl input double; st_CoorrSts input double; bool_ShtdwnAck input double; pPUD_st_AcChrgModeSt input double; pPUD_st_DcChrgModeSt input double; pPUD_st_AcHeatModeSt input double; pPUD_st_DcHeatModeSt input double; pPUD_st_DrvOnModeSt input double; s_ErrNoDrvON_na input double; AllowShutdownEpark_na input double; AllowShutdownVelocity_na input single; s_ErrNoAcHvChrg_na input double; pVMM_st_PUDCoorrReq output uint8; pVMM_st_CoorrSts output uint8; s_ErrNoDcHvChrg_na input double; s_ErrNoAcHvHeat_na input double; s_ErrNoDcHvHeat_na input double; s_ErrEmgHvOff_na input double; bool_restart local boolean; pVMM_st_MotCtlrModReq output uint8; s_ErrDrvOFF_na input double; s_ErrAcHvChrgOff_na input double; s_ErrDcHvChrgOff_na input double; s_ErrAcHvHeatOff_na input double; s_ErrDcHvHeatOff_na input double; pVMM_s_EparkShutdownTiOut_C input double; pVMM_kmph_VehLgtSpdThd_C input single; pVMM_s_ThermoShutdownTiOut_C input double; pVMM_s_ShtdwnAckDly_C input double; pVMM_s_EparkCheckTiOut_C input double
